simulink library "TECS"  (R2024a)
settings: Solver=VariableStepAuto  StartTime=0.0  StopTime=10.0  RelTol=1e-3
undefined symbols (not defined in the file): H0, PTCH_LIM_MAX_DEG, PTCH_LIM_MIN_DEG, TECS_CLMB_MAX, TECS_Freq, TECS_INTEG_GAIN, TECS_PTCH_DAMP, TECS_SINK_MIN, TECS_THR_DAMP, TECS_TIME_CONST, THR_TRIM, V0
settings Model: Creator=igmso  LastModifiedBy=igmso

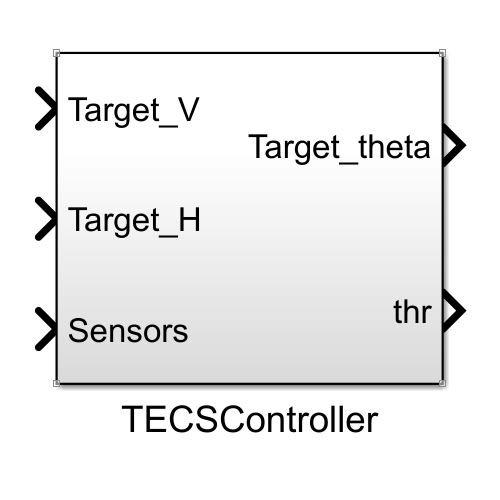
[thumbnail: Simulink's stored preview of the top-level diagram]
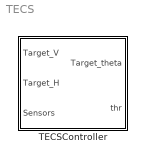
== system TECS ==
  TECSController : Subsystem

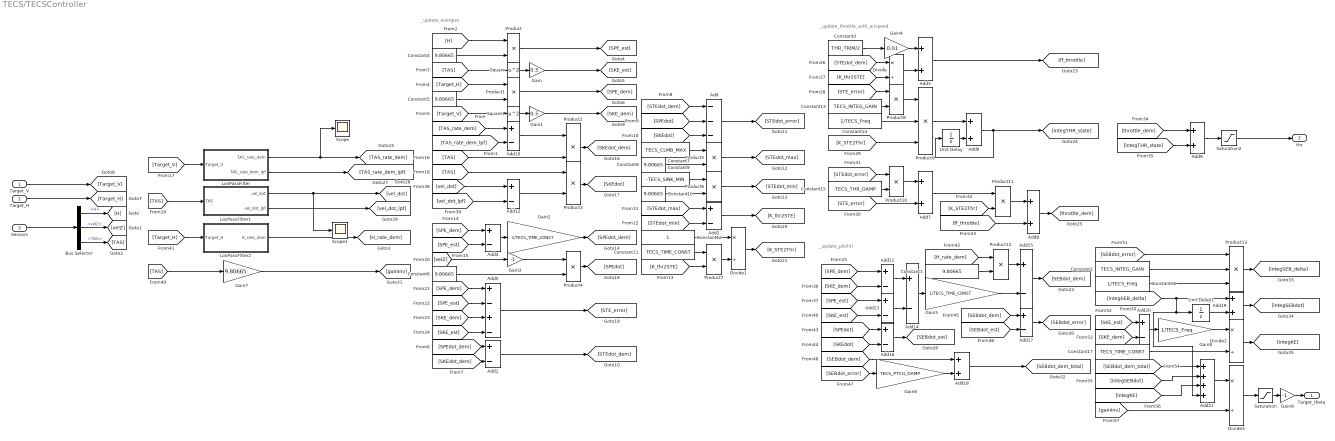
== system TECS/TECSController ==
  note: _update_pitch()
  note: _update_energies
  note: _update_throttle_with_airspeed
  Target_V : Inport  SampleTime=1/TECS_Freq
  Target_H : Inport  Port=2  SampleTime=1/TECS_Freq
  Sensors : Inport  Port=3  SampleTime=1/TECS_Freq
  Add : Sum  Inputs=---
  Add{1..2,4,10..17,20} (12 alike) : Sum  Inputs=+-
  Add{3,6..9,18..19} (7 alike) : Sum
  Add21 : Sum  Inputs=4
  Add5 : Sum  Inputs=+-+-
  Bus Selector : BusSelector  OutputSignals=H,velZ,TAS
  Constant{1,4..6,8,10} (6 alike) : Constant  Value=9.80665  SampleTime=1/TECS_Freq
  Constant11 : Constant  Value=TECS_TIME_CONST  SampleTime=1/TECS_Freq
  Constant12 : Constant  SampleTime=1/TECS_Freq
  Constant13 : Constant  Value=TECS_INTEG_GAIN  SampleTime=1/TECS_Freq
  Constant14 : Constant  Value=1/TECS_Freq  SampleTime=1/TECS_Freq
  Constant15 : Constant  Value=TECS_THR_DAMP  SampleTime=1/TECS_Freq
  Constant16 : Constant  Value=1/TECS_Freq  SampleTime=1/TECS_Freq
  Constant17 : Constant  Value=TECS_TIME_CONST  SampleTime=1/TECS_Freq
  Constant2 : Constant  Value=TECS_INTEG_GAIN  SampleTime=1/TECS_Freq
  Constant3 : Constant  Value=THR_TRIM/2  SampleTime=1/TECS_Freq
  Constant7 : Constant  Value=TECS_CLMB_MAX  SampleTime=1/TECS_Freq
  Constant9 : Constant  Value=-TECS_SINK_MIN  SampleTime=1/TECS_Freq
  Divide{,1..3} (4 alike) : Product  Inputs=*/
  Gain : Gain  Gain=0.5
  Gain1 : Gain  Gain=0.5
  Gain2 : Gain  Gain=1/TECS_TIME_CONST
  Gain3 : Gain  Gain=-1
  Gain4 : Gain  Gain=0.01
  Gain5 : Gain  Gain=1/TECS_TIME_CONST
  Gain6 : Gain  Gain=TECS_PTCH_DAMP
  Gain7 : Gain  Gain=9.80665
  Gain8 : Gain  Gain=1/TECS_Freq
  Gain9 : Gain  Gain=-1
  LosPassFilter : Subsystem
  LosPassFilter1 : Subsystem
  LosPassFilter2 : Subsystem
  Product{,1..6,8,10..12} (11 alike) : Product
  Product13 : Product  Inputs=3
  Product7 : Product  Inputs=**
  Product9 : Product  Inputs=3
  Saturation : Saturate  UpperLimit=deg2rad(PTCH_LIM_MAX_DEG)  LowerLimit=deg2rad(-PTCH_LIM_MIN_DEG)
  Saturation2 : Saturate  UpperLimit=1  LowerLimit=-1
  Scope : Scope
  Scope1 : Scope
  Square : Math  Operator=square
  Square1 : Math  Operator=square
  Unit Delay : UnitDelay  SampleTime=-1  StateName="\"integTHR_state\""  HasFrameUpgradeWarning=on
  Unit Delay1 : UnitDelay  SampleTime=-1  StateName="\"integTHR_state\""  HasFrameUpgradeWarning=on
  Target_theta : Outport
  thr : Outport  Port=2
  wires:
  Gain1/1 -> [SKE_dem]
  [SPEdot] -> Add/2
  [K_thr2STE] -> Product7/2
  Add2/1 -> [K_thr2STE]
  Add3/1 -> [ff_throttle]
  [STEdot_min] -> Add2/2
  [STEdot_max] -> Add2/1
  Product10/1 -> Add7/1
  [SPE_est] -> Add5/2
  Product7/1 -> Divide1/2
  [ff_throttle] -> Add8/2
  Constant12/1 -> Divide1/1
  Bus Selector/1 -> [H]  "<H>"
  [TAS] -> Product3/1
  Constant5/1 -> Product1/2
  Divide/1 -> Add3/2
  Constant8/1 -> Product5/2
  [SKEdot] -> Add/3
  Add9/1 -> Saturation2/1
  [STEdot_dem] -> Add/1
  Constant6/1 -> Product4/2
  Bus Selector/2 -> [velZ]  "<velZ>"
  [Target_V] -> Square1/1
  Product/1 -> [SPE_est]
  [SPE_est] -> Add4/2
  Add/1 -> [STEdot_error]
  Gain/1 -> [SKE_est]
  Product8/1 -> Product9/1
  Unit Delay/1 -> Add6/2
  Add7/1 -> Product11/1
  Constant10/1 -> Product6/2
  Square/1 -> Gain/1
  Constant4/1 -> Product/2
  [Target_H] -> Product1/1
  Constant15/1 -> Product10/2
  [H] -> Product/1
  Product9/1 -> Add6/1
  [K_STE2Thr] -> Product11/2
  Product3/1 -> [SKEdot]
  Constant11/1 -> Product7/1
  Add8/1 -> [throttle_dem]
  [SPEdot_dem] -> Add1/1
  [SKE_dem] -> Add5/3
  Product6/1 -> [STEdot_min]
  [K_thr2STE] -> Divide/2
  [STEdot_error] -> Product10/1
  [STE_error] -> Add7/2
  [TAS] -> Product2/2
  Add6/1 -> [integTHR_state], Unit Delay/1
  [STE_error] -> Product8/1
  [STEdot_dem] -> Divide/1
  Constant9/1 -> Product6/1
  Add4/1 -> Gain2/1
  Constant13/1 -> Product8/2
  [SKEdot_dem] -> Add1/2
  Product1/1 -> [SPE_dem]
  [TAS] -> Square/1
  Add5/1 -> [STE_error]
  [SPE_dem] -> Add5/1
  [integTHR_state] -> Add9/2
  Product5/1 -> [STEdot_max]
  Gain2/1 -> [SPEdot_dem]
  [SPE_dem] -> Add4/1
  Product4/1 -> [SPEdot]
  Bus Selector/3 -> [TAS]  "<TAS>"
  [throttle_dem] -> Add9/1
  Constant7/1 -> Product5/1
  Constant14/1 -> Product9/2
  [K_STE2Thr] -> Product9/3
  [SKE_est] -> Add5/4
  Constant3/1 -> Gain4/1
  Product11/1 -> Add8/1
  Add1/1 -> [STEdot_dem]
  Gain3/1 -> Product4/1
  [velZ] -> Gain3/1
  Square1/1 -> Gain1/1
  Target_V/1 -> [Target_V]
  Saturation2/1 -> thr/1
  Target_H/1 -> [Target_H]
  Sensors/1 -> Bus Selector/1
  [Target_V] -> LosPassFilter/1(Target_V)
  LosPassFilter/1(TAS_rate_dem) -> Scope/1, [TAS_rate_dem]
  LosPassFilter/2(TAS_rate_dem_lpf) -> [TAS_rate_dem_lpf]
  [TAS_rate_dem] -> Add10/1
  [TAS_rate_dem_lpf] -> Add10/2
  Add10/1 -> Product2/1
  Product2/1 -> [SKEdot_dem]
  Divide1/1 -> [K_STE2Thr]
  [TAS] -> LosPassFilter1/1(TAS)
  LosPassFilter1/2(vel_dot_lpf) -> [vel_dot_lpf]
  [vel_dot_lpf] -> Add12/2
  [vel_dot] -> Add12/1
  Add12/1 -> Product3/2
  LosPassFilter1/1(vel_dot) -> Scope1/1, [vel_dot]
  Gain4/1 -> Add3/1
  [SPE_dem] -> Add11/1
  [SKE_dem] -> Add11/2
  [SPE_est] -> Add13/1
  [SKE_est] -> Add13/2
  Add13/1 -> Add14/2
  Add11/1 -> Add14/1
  Add14/1 -> Gain5/1
  LosPassFilter2/1(H_rate_dem) -> [H_rate_dem]
  [Target_H] -> LosPassFilter2/1(Target_H)
  [H_rate_dem] -> Product12/1
  Constant1/1 -> Product12/2
  Product12/1 -> Add15/1
  Gain5/1 -> Add15/2
  Add15/1 -> [SEBdot_dem]
  [SPEdot] -> Add16/1
  [SKEdot] -> Add16/2
  Add16/1 -> [SEBdot_est]
  [SEBdot_dem] -> Add17/1
  [SEBdot_est] -> Add17/2
  Add17/1 -> [SEBdot_error]
  [SEBdot_error] -> Gain6/1
  Gain6/1 -> Add18/2
  [SEBdot_dem] -> Add18/1
  [TAS] -> Gain7/1
  Gain7/1 -> [gainInv]
  Add18/1 -> [SEBdot_dem_total]
  Constant16/1 -> Product13/3
  Constant2/1 -> Product13/2
  [SEBdot_error] -> Product13/1
  Product13/1 -> [integSEB_delta]
  [integSEB_delta] -> Add21/4, Unit Delay1/1, Add19/1
  Unit Delay1/1 -> Add19/2
  Add19/1 -> [integSEBdot]
  [SKE_est] -> Add20/1
  [SKE_dem] -> Add20/2
  Add20/1 -> Gain8/1
  Gain8/1 -> Divide2/1
  Constant17/1 -> Divide2/2
  Divide2/1 -> [integKE]
  [integSEBdot] -> Add21/2
  [SEBdot_dem_total] -> Add21/1
  [integKE] -> Add21/3
  Add21/1 -> Divide3/1
  [gainInv] -> Divide3/2
  Divide3/1 -> Saturation/1
  Saturation/1 -> Gain9/1
  Gain9/1 -> Target_theta/1

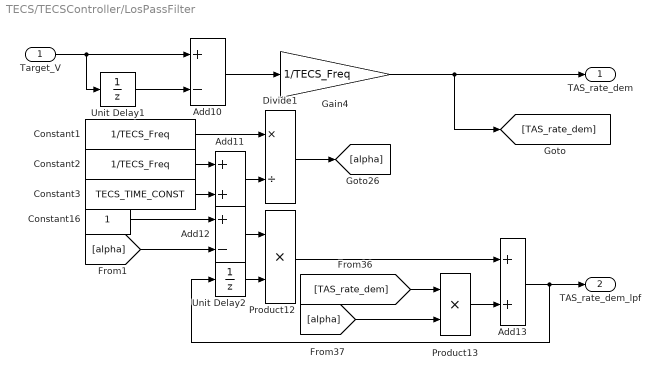
== system TECS/TECSController/LosPassFilter ==
  Target_V : Inport
  Add10 : Sum  Inputs=+-
  Add11 : Sum
  Add12 : Sum  Inputs=+-
  Add13 : Sum
  Constant1 : Constant  Value=1/TECS_Freq  SampleTime=1/TECS_Freq
  Constant16 : Constant  SampleTime=1/TECS_Freq
  Constant2 : Constant  Value=1/TECS_Freq  SampleTime=1/TECS_Freq
  Constant3 : Constant  Value=TECS_TIME_CONST  SampleTime=1/TECS_Freq
  Divide1 : Product  Inputs=*/
  Gain4 : Gain  Gain=1/TECS_Freq
  Product12 : Product
  Product13 : Product
  Unit Delay1 : UnitDelay  InitialCondition=V0  SampleTime=-1  HasFrameUpgradeWarning=on
  Unit Delay2 : UnitDelay  SampleTime=-1  HasFrameUpgradeWarning=on
  TAS_rate_dem : Outport
  TAS_rate_dem_lpf : Outport  Port=2
  wires:
  [alpha] -> Product13/2
  Constant3/1 -> Add11/2
  Product13/1 -> Add13/2
  [TAS_rate_dem] -> Product13/1
  Constant2/1 -> Add11/1
  Add11/1 -> Divide1/2
  Divide1/1 -> [alpha]
  Constant1/1 -> Divide1/1
  Add10/1 -> Gain4/1
  Add12/1 -> Product12/1
  [alpha] -> Add12/2
  Constant16/1 -> Add12/1
  Add13/1 -> TAS_rate_dem_lpf/1, Unit Delay2/1
  Product12/1 -> Add13/1
  Unit Delay2/1 -> Product12/2
  Unit Delay1/1 -> Add10/2
  Target_V/1 -> Unit Delay1/1, Add10/1
  Gain4/1 -> [TAS_rate_dem], TAS_rate_dem/1

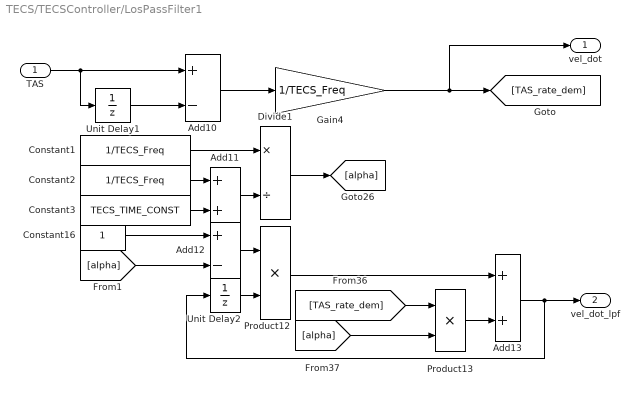
== system TECS/TECSController/LosPassFilter1 ==
  TAS : Inport
  Add10 : Sum  Inputs=+-
  Add11 : Sum
  Add12 : Sum  Inputs=+-
  Add13 : Sum
  Constant1 : Constant  Value=1/TECS_Freq  SampleTime=1/TECS_Freq
  Constant16 : Constant  SampleTime=1/TECS_Freq
  Constant2 : Constant  Value=1/TECS_Freq  SampleTime=1/TECS_Freq
  Constant3 : Constant  Value=TECS_TIME_CONST  SampleTime=1/TECS_Freq
  Divide1 : Product  Inputs=*/
  Gain4 : Gain  Gain=1/TECS_Freq
  Product12 : Product
  Product13 : Product
  Unit Delay1 : UnitDelay  InitialCondition=V0  SampleTime=-1  HasFrameUpgradeWarning=on
  Unit Delay2 : UnitDelay  SampleTime=-1  HasFrameUpgradeWarning=on
  vel_dot : Outport
  vel_dot_lpf : Outport  Port=2
  wires:
  Gain4/1 -> vel_dot/1, [TAS_rate_dem]
  TAS/1 -> Unit Delay1/1, Add10/1
  Unit Delay1/1 -> Add10/2
  Unit Delay2/1 -> Product12/2
  Product12/1 -> Add13/1
  Add13/1 -> Unit Delay2/1, vel_dot_lpf/1
  Constant16/1 -> Add12/1
  [alpha] -> Add12/2
  Add12/1 -> Product12/1
  Add10/1 -> Gain4/1
  Constant1/1 -> Divide1/1
  Divide1/1 -> [alpha]
  Add11/1 -> Divide1/2
  Constant2/1 -> Add11/1
  [TAS_rate_dem] -> Product13/1
  Product13/1 -> Add13/2
  Constant3/1 -> Add11/2
  [alpha] -> Product13/2

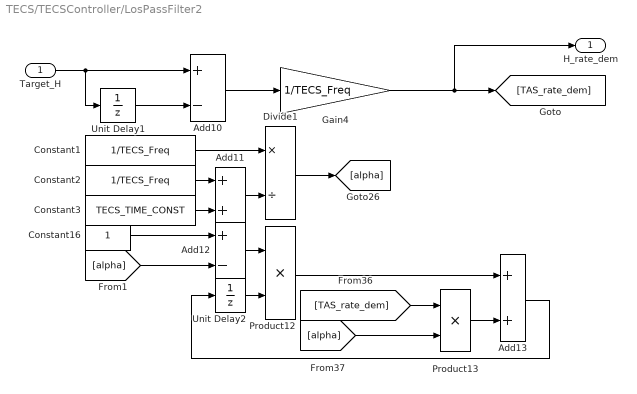
== system TECS/TECSController/LosPassFilter2 ==
  Target_H : Inport
  Add10 : Sum  Inputs=+-
  Add11 : Sum
  Add12 : Sum  Inputs=+-
  Add13 : Sum
  Constant1 : Constant  Value=1/TECS_Freq  SampleTime=1/TECS_Freq
  Constant16 : Constant  SampleTime=1/TECS_Freq
  Constant2 : Constant  Value=1/TECS_Freq  SampleTime=1/TECS_Freq
  Constant3 : Constant  Value=TECS_TIME_CONST  SampleTime=1/TECS_Freq
  Divide1 : Product  Inputs=*/
  Gain4 : Gain  Gain=1/TECS_Freq
  Product12 : Product
  Product13 : Product
  Unit Delay1 : UnitDelay  InitialCondition=H0  SampleTime=-1  HasFrameUpgradeWarning=on
  Unit Delay2 : UnitDelay  SampleTime=-1  HasFrameUpgradeWarning=on
  H_rate_dem : Outport
  wires:
  [alpha] -> Product13/2
  Constant3/1 -> Add11/2
  Product13/1 -> Add13/2
  [TAS_rate_dem] -> Product13/1
  Constant2/1 -> Add11/1
  Add11/1 -> Divide1/2
  Divide1/1 -> [alpha]
  Constant1/1 -> Divide1/1
  Add10/1 -> Gain4/1
  Add12/1 -> Product12/1
  [alpha] -> Add12/2
  Constant16/1 -> Add12/1
  Add13/1 -> Unit Delay2/1
  Product12/1 -> Add13/1
  Unit Delay2/1 -> Product12/2
  Unit Delay1/1 -> Add10/2
  Target_H/1 -> Add10/1, Unit Delay1/1
  Gain4/1 -> [TAS_rate_dem], H_rate_dem/1
